simulink model "CntrlBaseline"  (R2016b)
settings: Solver=FixedStepAuto  StartTime=0.0  StopTime=10.0  RelTol=1e-3  SampleTimeConstraint=STIndependent
undefined symbols (not defined in the file): AC, MPCSampleTime, pitch_gains, roll_gains, TrimCondition, yaw_damper_den, yaw_damper_num
settings Model: Creator=UAVLAB  LastModifiedBy=UAVLAB

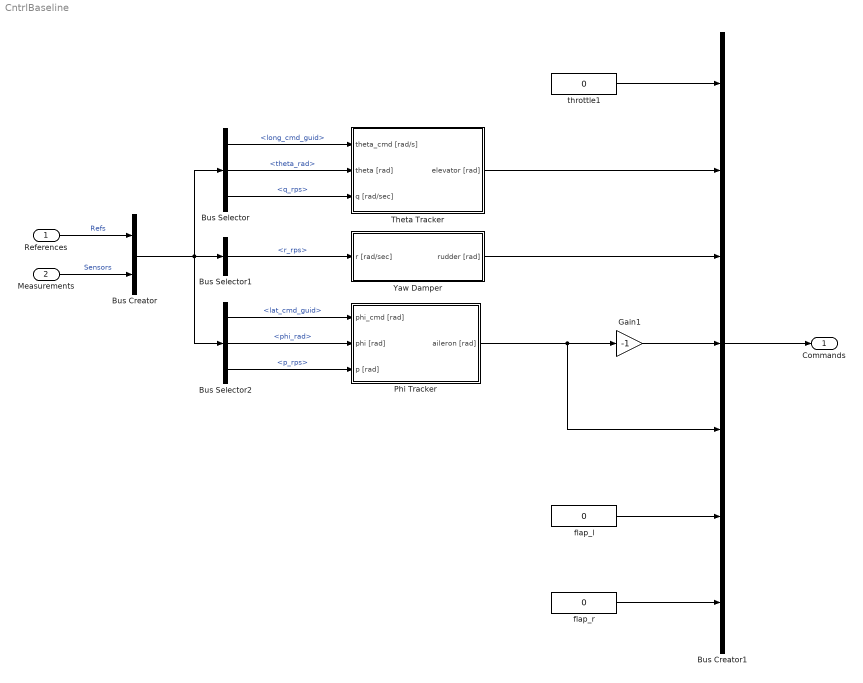
== system CntrlBaseline ==
  References : Inport  OutDataTypeStr=Bus: Refs
  Measurements : Inport  Port=2  OutDataTypeStr=Bus: Sensors
  Bus Creator1 : BusCreator  Inputs=7  OutDataTypeStr=Bus: Commands
      settings: InheritFromInputs=off
  Bus Creator : BusCreator  Inputs=2
  Bus Selector : BusSelector  OutputSignals=Refs.long_cmd_guid,Sensors.theta_rad,Sensors.q_rps
  Bus Selector1 : BusSelector  OutputSignals=Sensors.r_rps
  Bus Selector2 : BusSelector  OutputSignals=Refs.lat_cmd_guid,Sensors.phi_rad,Sensors.p_rps
  Gain1 : Gain  Gain=-1
  Phi Tracker : Subsystem
  Theta Tracker : Subsystem
  Yaw Damper : Subsystem
  flap_l : Constant  Value=0  SampleTime=-1
  flap_r : Constant  Value=0  SampleTime=-1
  throttle1 : Constant  Value=0  SampleTime=-1
  Commands : Outport  OutDataTypeStr=Bus: Commands
  wires:
  Bus Selector/1 -> Theta Tracker/1(theta_cmd [rad/s])  "<long_cmd_guid>"
  Bus Creator1/1 -> Commands/1
  flap_l/1 -> Bus Creator1/6
  Measurements/1 -> Bus Creator/2  "Sensors"
  flap_r/1 -> Bus Creator1/7
  throttle1/1 -> Bus Creator1/1
  Yaw Damper/1(rudder [rad]) -> Bus Creator1/3
  Theta Tracker/1(elevator [rad]) -> Bus Creator1/2
  Bus Selector2/1 -> Phi Tracker/1(phi_cmd [rad])  "<lat_cmd_guid>"
  Bus Selector1/1 -> Yaw Damper/1(r [rad/sec])  "<r_rps>"
  References/1 -> Bus Creator/1  "Refs"
  Bus Selector2/3 -> Phi Tracker/3(p [rad])  "<p_rps>"
  Bus Selector/3 -> Theta Tracker/3(q [rad/sec])  "<q_rps>"
  Bus Creator/1 -> Bus Selector2/1, Bus Selector/1, Bus Selector1/1
  Bus Selector/2 -> Theta Tracker/2(theta [rad])  "<theta_rad>"
  Bus Selector2/2 -> Phi Tracker/2(phi [rad])  "<phi_rad>"
  Phi Tracker/1(aileron [rad]) -> Bus Creator1/5, Gain1/1
  Gain1/1 -> Bus Creator1/4

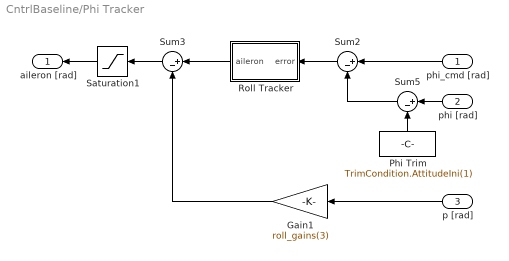
== system CntrlBaseline/Phi Tracker ==
  phi_cmd [rad] : Inport
  phi [rad] : Inport  Port=2
  p [rad] : Inport  Port=3
  Gain1 : Gain  Gain=roll_gains(3)
  Phi Trim : Constant  Value=TrimCondition.AttitudeIni(1)  SampleTime=-1
  Roll Tracker : Subsystem
  Saturation1 : Saturate  UpperLimit=AC.Actuator.r_aileron.PosLim-TrimCondition.Inputs.Actuator(3)*.5  LowerLimit=AC.Actuator.r_aileron.NegLim-TrimCondition.Inputs.Actuator(3)*.5
  Sum2 : Sum  Inputs=|+-
  Sum3 : Sum  Inputs=|+-
  Sum5 : Sum  Inputs=|+-
  aileron [rad] : Outport
  wires:
  phi_cmd [rad]/1 -> Sum2/1
  Gain1/1 -> Sum3/2
  p [rad]/1 -> Gain1/1
  Sum3/1 -> Saturation1/1
  Sum2/1 -> Roll Tracker/1(error)
  Phi Trim/1 -> Sum5/2
  Sum5/1 -> Sum2/2
  phi [rad]/1 -> Sum5/1
  Saturation1/1 -> aileron [rad]/1
  Roll Tracker/1(aileron) -> Sum3/1

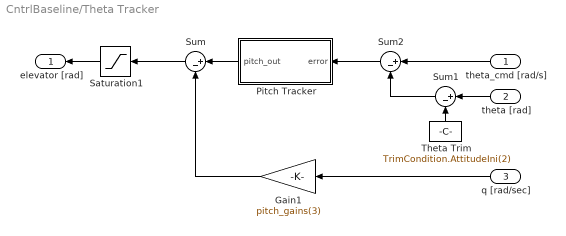
== system CntrlBaseline/Theta Tracker ==
  theta_cmd [rad/s] : Inport
  theta [rad] : Inport  Port=2
  q [rad/sec] : Inport  Port=3
  " Theta Trim" : Constant  Value=TrimCondition.AttitudeIni(2)  SampleTime=-1
  Gain1 : Gain  Gain=pitch_gains(3)
  Pitch Tracker : Subsystem
  Saturation1 : Saturate  UpperLimit=AC.Actuator.elevator.PosLim-TrimCondition.Inputs.Actuator(1)  LowerLimit=AC.Actuator.elevator.NegLim-TrimCondition.Inputs.Actuator(1)
  Sum : Sum  Inputs=|+-
  Sum1 : Sum  Inputs=|+-
  Sum2 : Sum  Inputs=|+-
  elevator [rad] : Outport
  wires:
  Gain1/1 -> Sum/2
  q [rad/sec]/1 -> Gain1/1
  Sum/1 -> Saturation1/1
  Pitch Tracker/1(pitch_out) -> Sum/1
  theta_cmd [rad/s]/1 -> Sum2/1
  theta [rad]/1 -> Sum1/1
  " Theta Trim"/1 -> Sum1/2
  Sum1/1 -> Sum2/2
  Saturation1/1 -> elevator [rad]/1
  Sum2/1 -> Pitch Tracker/1(error)

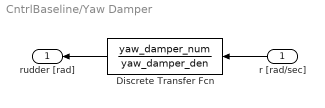
== system CntrlBaseline/Yaw Damper ==
  r [rad/sec] : Inport
  Discrete Transfer Fcn : DiscreteTransferFcn  Numerator=yaw_damper_num  Denominator=yaw_damper_den
  rudder [rad] : Outport
  wires:
  r [rad/sec]/1 -> Discrete Transfer Fcn/1
  Discrete Transfer Fcn/1 -> rudder [rad]/1

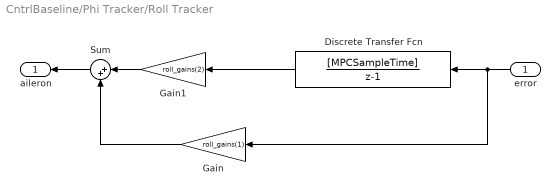
== system CntrlBaseline/Phi Tracker/Roll Tracker ==
  error : Inport
  Discrete Transfer Fcn : DiscreteTransferFcn  Numerator=[MPCSampleTime]  Denominator=[1 -1]
  Gain : Gain  Gain=roll_gains(1)
  Gain1 : Gain  Gain=roll_gains(2)
  Sum : Sum  Inputs=|++
  aileron : Outport
  wires:
  Gain1/1 -> Sum/1
  Sum/1 -> aileron/1
  Gain/1 -> Sum/2
  error/1 -> Discrete Transfer Fcn/1, Gain/1
  Discrete Transfer Fcn/1 -> Gain1/1

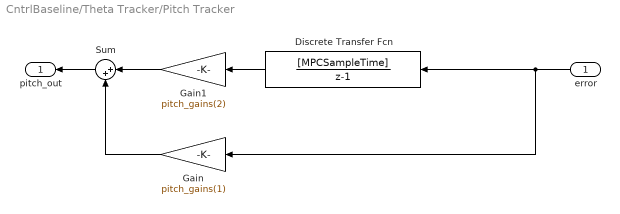
== system CntrlBaseline/Theta Tracker/Pitch Tracker ==
  error : Inport
  Discrete Transfer Fcn : DiscreteTransferFcn  Numerator=[MPCSampleTime]  Denominator=[1 -1]
  Gain : Gain  Gain=pitch_gains(1)
  Gain1 : Gain  Gain=pitch_gains(2)
  Sum : Sum  Inputs=|++
  pitch_out : Outport
  wires:
  Discrete Transfer Fcn/1 -> Gain1/1
  Gain1/1 -> Sum/1
  Sum/1 -> pitch_out/1
  Gain/1 -> Sum/2
  error/1 -> Gain/1, Discrete Transfer Fcn/1
